simulink model "RampFunc"  (R2023b)
settings: Solver=FixedStepDiscrete  StartTime=0.0  StopTime=10.0  FixedStep=0.001  RelTol=1e-3
settings Model: Creator=win  LastModifiedBy=win

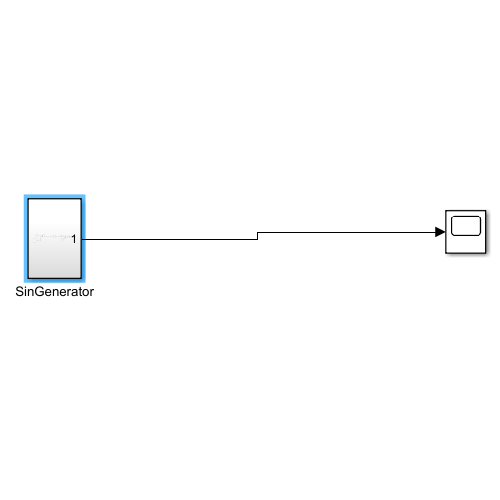
[thumbnail: Simulink's stored preview of the top-level diagram]
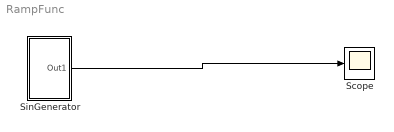
== system RampFunc ==
  Scope : Scope
  SinGenerator : Subsystem
  wires:
  SinGenerator/1(Out1) -> Scope/1

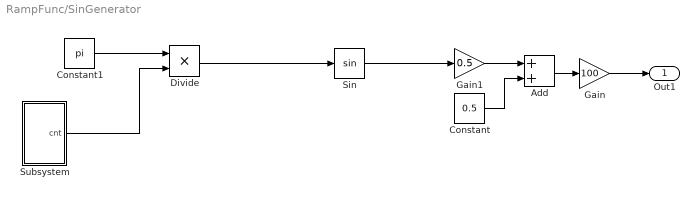
== system RampFunc/SinGenerator ==
  Add : Sum
  Constant : Constant  Value=0.5
  Constant1 : Constant  Value=pi  OutDataTypeStr=single
  Divide : Product  Inputs=**  OutDataTypeStr=single
  Gain : Gain  Gain=100
  Gain1 : Gain  Gain=0.5
  Sin : Trigonometry
  Subsystem : Subsystem  mask{trsh=2, stp=0.01}
      mask prompts: trsh "Treshold"; stp "Step"
  Out1 : Outport
  wires:
  Gain/1 -> Out1/1
  Divide/1 -> Sin/1
  Sin/1 -> Gain1/1
  Gain1/1 -> Add/1
  Add/1 -> Gain/1
  Constant/1 -> Add/2
  Constant1/1 -> Divide/1
  Subsystem/1(cnt) -> Divide/2

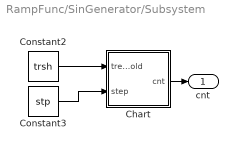
== system RampFunc/SinGenerator/Subsystem ==
  Chart : Stateflow chart  TreatAsAtomicUnit=on
  Constant2 : Constant  Value=trsh
  Constant3 : Constant  Value=stp
  cnt : Outport
  wires:
  Constant2/1 -> Chart/1(treshold)
  Chart/1(cnt) -> cnt/1
  Constant3/1 -> Chart/2(step)

== stateflow chart RampFunc/SinGenerator/Subsystem/Chart ==
  state RESET
    cnt =0;
  state IDLE
    cnt = cnt + step;
  (default) -> RESET
  RESET -> IDLE : [cnt ==0]
  IDLE -> RESET : [cnt>=treshold]
  data: treshold input; step input; cnt output
